simulink model "example_model"  (R2018b)
settings: Solver=FixedStepAuto  StartTime=0.0  StopTime=Inf  FixedStep=.1  RelTol=1e-3  EnableMultiTasking=on
model workspace (MAT data in the model file):
  SL_ROS_VariableLengthArrays_MaxSizes.CommonInfo.ArrayTruncateAction = 'EmitWarning'
  SL_ROS_VariableLengthArrays_MaxSizes.MsgTypeMap = containers.Map
  SL_ROS_VariableLengthArrays_MaxSizes.MsgTypeMap.serialization.keys = {'sensor_msgs/LaserScan'}
  SL_ROS_VariableLengthArrays_MaxSizes.MsgTypeMap.serialization.values{1}(1).PropertyName = 'Intensities'
  SL_ROS_VariableLengthArrays_MaxSizes.MsgTypeMap.serialization.values{1}(1).DataType = 'single'
  SL_ROS_VariableLengthArrays_MaxSizes.MsgTypeMap.serialization.values{1}(1).MaxLength = 350
  SL_ROS_VariableLengthArrays_MaxSizes.MsgTypeMap.serialization.values{1}(2).PropertyName = 'Ranges'
  SL_ROS_VariableLengthArrays_MaxSizes.MsgTypeMap.serialization.values{1}(2).DataType = 'single'
  SL_ROS_VariableLengthArrays_MaxSizes.MsgTypeMap.serialization.values{1}(2).MaxLength = 350
  SL_ROS_VariableLengthArrays_MaxSizes.MsgTypeMap.serialization.uniformity = 0
  SL_ROS_VariableLengthArrays_MaxSizes.MsgTypeMap.serialization.keyType = 'char'
  SL_ROS_VariableLengthArrays_MaxSizes.MsgTypeMap.serialization.valueType = 'any'
undefined symbols (not defined in the file): FifthOutput, MotorOutput, SteerOutput
libraries: robotlib x5
settings Model: Creator=nate  LastModifiedBy=nate
settings SolverCC: PositivePriorityOrder=on
settings OptimizationCC: EnhancedBackFolding=on  PassReuseOutputArgsAs=Individual arguments  MaxStackSize=64  OptimizeBlockOrder=speed  DifferentSizesBufferReuse=on  OptimizationCustomize=off
settings DebuggingCC: ParameterTunabilityLossMsg=error
settings HardwareCC: ProdBitPerPointer=32  ProdBitPerSizeT=32  ProdBitPerPtrDiffT=32  ProdLargestAtomicInteger=Long  ProdLargestAtomicFloat=Double  ProdWordSize=32  ProdHWDeviceType=ARM Compatible->ARM Cortex  TargetLargestAtomicInteger=Long  TargetLargestAtomicFloat=Double  TargetIntDivRoundTo=Zero  TargetEndianess=LittleEndian  TargetHWDeviceType=ARM Compatible->ARM Cortex  ProdEqTarget=off
settings SFSimCC: MATLABDynamicMemAlloc=off
settings RTWCC: SystemTargetFile=ert.tlc  HardwareBoard=Raspberry Pi - Robot Operating System (ROS)  TLCOptions="-aInlineSetEventsForThisBaseRateFcn=TLC_FALSE -aSuppressMultiTaskScheduler=TLC_FALSE  -aRateBasedStepFcn=0"  GenCodeOnly=on  TemplateMakefile=ert_default_tmf  GenerateReport=on  Toolchain=Catkin  IncludeHyperlinkInReport=on  LaunchReport=on  TargetLang=C++  GenerateTraceInfo=on  GenerateTraceReport=on  GenerateTraceReportSl=on  GenerateTraceReportSf=on  GenerateTraceReportEml=on  CheckMdlBeforeBuild=Warning
settings CodeAppCC: ForceParamTrailComments=on  IgnoreCustomStorageClasses=off  OperatorAnnotations=on  SimulinkDataObjDesc=on  SFDataObjDesc=on  InsertBlockDesc=on
settings ERTTargetCC: SupportVariableSizeSignals=on  ExtMode=on

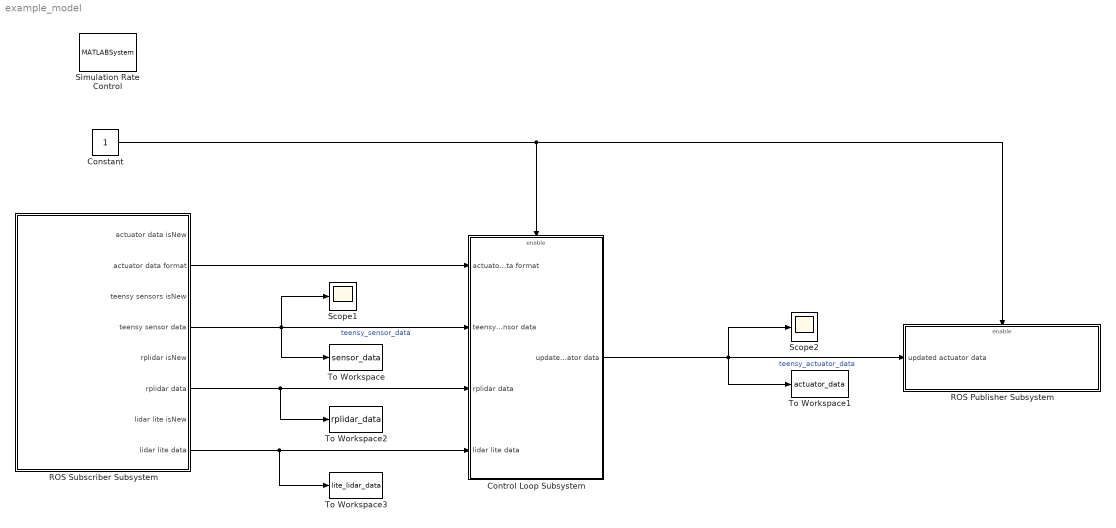
== system example_model ==
  Constant : Constant
  Control Loop Subsystem : Subsystem
  "ROS Publisher Subsystem " : Subsystem
  ROS Subscriber Subsystem : Subsystem
  Scope1 : Scope
  Scope2 : Scope
  Simulation Rate Control : MATLABSystem  System=ExampleHelperSimulationRateControl  SampleTime=.05
      mask Type: ExampleHelperSimulationRateControl
      mask Display: disp('Rate Control');
  To Workspace : ToWorkspace  VariableName=sensor_data  SaveFormat=Timeseries  SampleTime=-1
  To Workspace1 : ToWorkspace  VariableName=actuator_data  SaveFormat=Timeseries  SampleTime=-1
  To Workspace2 : ToWorkspace  VariableName=rplidar_data  SaveFormat=Timeseries  SampleTime=-1
  To Workspace3 : ToWorkspace  VariableName=lite_lidar_data  SaveFormat=Timeseries  SampleTime=-1
  wires:
  ROS Subscriber Subsystem/2(actuator data format) -> Control Loop Subsystem/1(actuator data format)
  ROS Subscriber Subsystem/4("teensy sensor data ") -> To Workspace/1, Scope1/1, Control Loop Subsystem/2(teensy sensor data)  "teensy_sensor_data"
  Control Loop Subsystem/1(updated actuator data) -> To Workspace1/1, Scope2/1, "ROS Publisher Subsystem "/1(updated actuator data)  "teensy_actuator_data"
  Constant/1 -> "ROS Publisher Subsystem "/Enable, Control Loop Subsystem/Enable
  ROS Subscriber Subsystem/6(rplidar data) -> To Workspace2/1, Control Loop Subsystem/3(rplidar data)
  ROS Subscriber Subsystem/8(lidar lite data) -> To Workspace3/1, Control Loop Subsystem/4(lidar lite data)

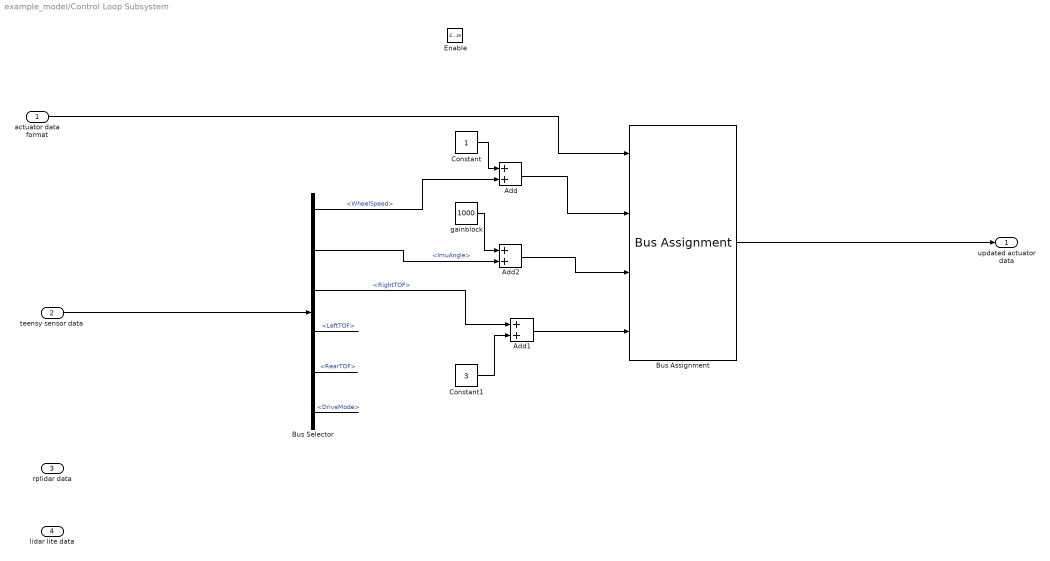
== system example_model/Control Loop Subsystem ==
  actuator data format : Inport
  teensy sensor data : Inport  Port=2
  rplidar data : Inport  Port=3
  lidar lite data : Inport  Port=4
  Enable : EnablePort
  Add : Sum
  Add1 : Sum
  Add2 : Sum  OutDataTypeStr=int16
  Bus Assignment : BusAssignment  AssignedSignals=MotorOutput,SteerOutput,FifthOutput
  Bus Selector : BusSelector  OutputSignals=WheelSpeed,ImuAngle,RightTOF,LeftTOF,RearTOF,DriveMode
  Constant : Constant  OutDataTypeStr=int16
  Constant1 : Constant  Value=3  OutDataTypeStr=int16
  gainblock : Constant  Value=1000  OutDataTypeStr=int16
  updated actuator data : Outport
  wires:
  Add1/1 -> Bus Assignment/4
  Add/1 -> Bus Assignment/2
  teensy sensor data/1 -> Bus Selector/1
  Bus Selector/3 -> Add1/1  "<RightTOF>"
  Constant1/1 -> Add1/2
  Bus Selector/2 -> Add2/2  "<ImuAngle>"
  Add2/1 -> Bus Assignment/3
  Bus Selector/1 -> Add/2  "<WheelSpeed>"
  actuator data format/1 -> Bus Assignment/1
  gainblock/1 -> Add2/1
  Constant/1 -> Add/1
  Bus Assignment/1 -> updated actuator data/1
  Bus Selector/4 -> ?  "<LeftTOF>"
  Bus Selector/5 -> ?  "<RearTOF>"
  Bus Selector/6 -> ?  "<DriveMode>"

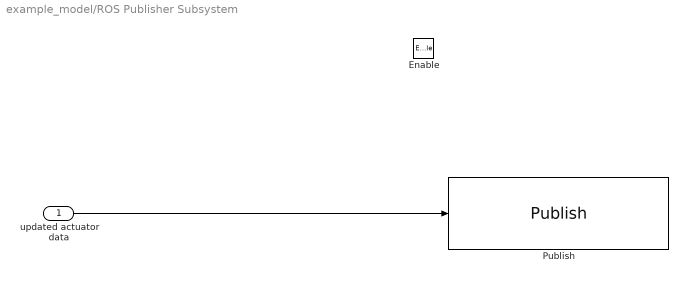
== system example_model/ROS Publisher Subsystem  ==
  updated actuator data : Inport
  Enable : EnablePort
  Publish : robotlib/Publish  topicSource=Select from ROS network  topic=/pi_comm_node/teensy_actuator_data  messageType=semi_truck/Teensy_Actuators  messageQueueLength=1
      link override SinkBlock: ROSTopic=/pi_comm_node/teensy_actuator_data  ROSMessageType=semi_truck/Teensy_Actuators  SLBusName=SL_Bus_myROScomm_semi_truck_Teensy_Actuators  ModelName=myROScomm  BlockId=Pub_myROScomm_9
      settings: SourceProductBaseCode=RO
  wires:
  updated actuator data/1 -> Publish/1

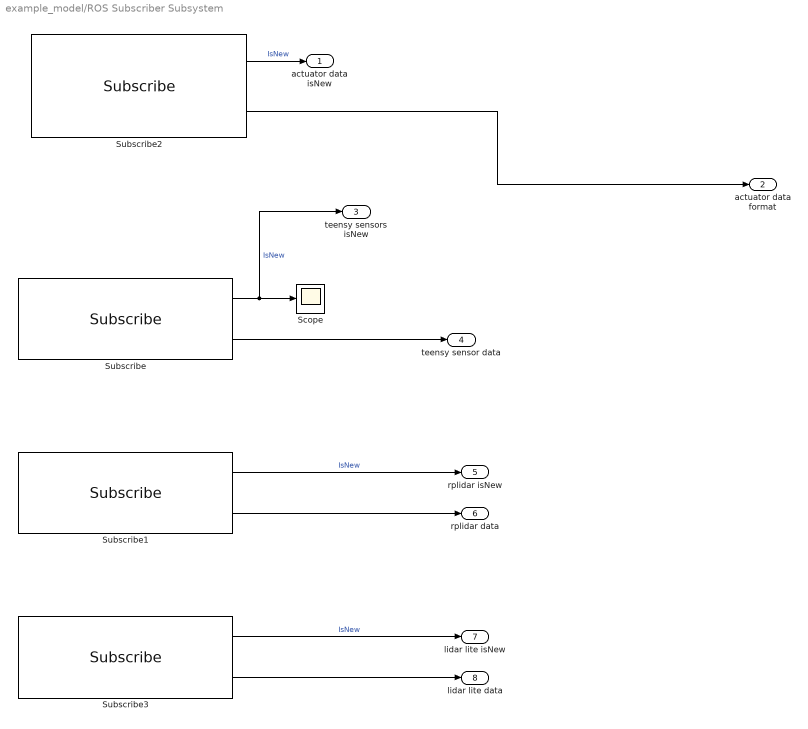
== system example_model/ROS Subscriber Subsystem ==
  Scope : Scope
  Subscribe : robotlib/Subscribe  topicSource=Select from ROS network  topic=/pi_comm_node/teensy_sensor_data  messageType=semi_truck/Teensy_Sensors  sampleTime=-1  messageQueueLength=51
      settings: SourceProductBaseCode=RO
  Subscribe1 : robotlib/Subscribe  topicSource=Select from ROS network  topic=/scan_rplidar  messageType=sensor_msgs/LaserScan  sampleTime=-1  messageQueueLength=51
      settings: SourceProductBaseCode=RO
  Subscribe2 : robotlib/Subscribe  topicSource=Select from ROS network  topic=/pi_comm_node/teensy_actuator_data  messageType=semi_truck/Teensy_Actuators  sampleTime=-1  messageQueueLength=51
      settings: SourceProductBaseCode=RO
  Subscribe3 : robotlib/Subscribe  topicSource=Select from ROS network  topic=/scan_lidar_lite  messageType=sensor_msgs/LaserScan  sampleTime=-1  messageQueueLength=51
      settings: SourceProductBaseCode=RO
  actuator data isNew : Outport
  actuator data format : Outport  Port=2
  "teensy sensors isNew " : Outport  Port=3
  "teensy sensor data " : Outport  Port=4
  "rplidar isNew " : Outport  Port=5
  rplidar data : Outport  Port=6
  "lidar lite isNew " : Outport  Port=7
  lidar lite data : Outport  Port=8
  wires:
  Subscribe2/1 -> actuator data isNew/1  "IsNew"
  Subscribe/1 -> "teensy sensors isNew "/1, Scope/1  "IsNew"
  Subscribe2/2 -> actuator data format/1
  Subscribe/2 -> "teensy sensor data "/1
  Subscribe1/2 -> rplidar data/1
  Subscribe1/1 -> "rplidar isNew "/1  "IsNew"
  Subscribe3/1 -> "lidar lite isNew "/1  "IsNew"
  Subscribe3/2 -> lidar lite data/1
